simulink model "sim_y"  (R2019b)
settings: Solver=VariableStepAuto  StartTime=0.0  StopTime=10.0  RelTol=1e-3
settings Model: Creator=vidma  LastModifiedBy=vidma

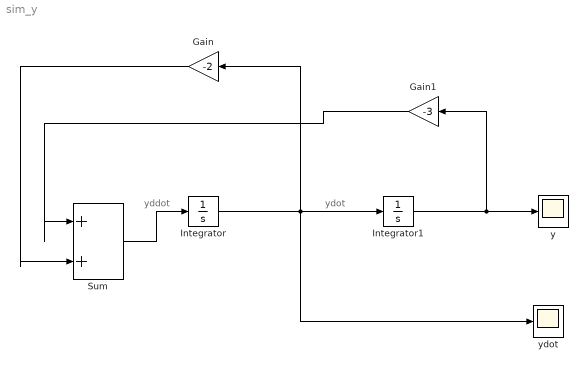
== system sim_y ==
  note: ydot
  note: yddot
  Gain : Gain  Gain=-2
  Gain1 : Gain  Gain=-3
  Integrator : Integrator
  Integrator1 : Integrator  InitialCondition=1
  Sum : Sum  Inputs=|++
  y : Scope
  ydot : Scope
  wires:
  Integrator1/1 -> Gain1/1, y/1
  Sum/1 -> Integrator/1
  Gain1/1 -> Sum/1
  Gain/1 -> Sum/2
  Integrator/1 -> ydot/1, Gain/1, Integrator1/1
